simulink library "AEMS_Standard_Library"  (R2016b)
settings: Solver=ode45  StartTime=0.0  StopTime=10.0  RelTol=1e-3
undefined symbols (not defined in the file or in its folder): BkPY, carto, Cbx_extegr, Cbx_lpegrsys, Cbx_portegr, Cnx_bnk_nr_conf, Cnx_cyl_nr_conf, ConfigManagement, configuration_management, Cxx_dcm_io_tmr_end_xxxx, Cxx_dcm_rt_tmr_end, Cxx_DID_xxxx_IO_max, Cxx_DID_xxxx_IO_min, Cxx_egrhsofs, Cxx_vmaniegi, DEM_DEBOUNCE_FREEZE, DEM_DTR_CTL_INVISIBLE, DEM_DTR_CTL_NORMAL, Dem_DtrId2_XXX, Dem_DtrId3_XXX, Dem_DtrId4_XXX, Dem_DtrId5_XXX, Dem_DtrId6_XXX, Dem_DtrId7_XXX, Dem_DtrId8_XXX, Dem_DtrId9_XXX, Dem_DtrId_XXX, Dem_EnableConditionId2_XXX, Dem_EnableConditionId3_XXX, Dem_EnableConditionId4_XXX, Dem_EnableConditionId5_XXX, Dem_EnableConditionId6_XXX, Dem_EnableConditionId7_XXX, Dem_EnableConditionId8_XXX, Dem_EnableConditionId_XXX, Dem_EventId, Dem_EventId2_XXX, Dem_EventId3_XXX, Dem_EventId4_XXX, Dem_EventId5_XXX, Dem_EventId6_XXX, Dem_EventId7_XXX, Dem_EventId8_XXX, Dem_EventId9_XXX, Dem_EventId_Device_Faulttype, Dem_EventId_XXX, DEM_IUMPR_GENERAL_DENOMINATOR, DEM_OPCYC_IGNITION, Dem_RatioId2_XXX, Dem_RatioId3_XXX, Dem_RatioId4_XXX, Dem_RatioId5_XXX, Dem_RatioId6_XXX, Dem_RatioId7_XXX, Dem_RatioId8_XXX, Dem_RatioId_XXX, Dem_StorageConditionId2_XXX, Dem_StorageConditionId3_XXX, Dem_StorageConditionId4_XXX, Dem_StorageConditionId5_XXX ... (+65)
libraries: AEMS_Standard_Library x477, simulink x2
(part 25 of 39)

== system AEMS_Standard_Library/SUB/AEMS_DEM_TIME_BASED_DEBOUNCE_THRSHOLD_DYN_6D ==
  note: DemDebounceBehavior
  flag_set : Inport
  conditionfulfilled : Inport  Port=2
  prefailed : Inport  Port=3
  prepassed : Inport  Port=4
  reseteventdebounce : Inport  Port=5
  failedthreshold : Inport  Port=6
  passedthreshold : Inport  Port=7
  AEMS_DEM_TIME_BASED_DEBOUNCE_THRSHOLD_DYN_CALL1 : Subsystem
  AEMS_DEM_TIME_BASED_DEBOUNCE_THRSHOLD_DYN_CALL2 : Subsystem
  AEMS_DEM_TIME_BASED_DEBOUNCE_THRSHOLD_DYN_CALL3 : Subsystem
  AEMS_DEM_TIME_BASED_DEBOUNCE_THRSHOLD_DYN_CALL4 : Subsystem
  AEMS_DEM_TIME_BASED_DEBOUNCE_THRSHOLD_DYN_CALL5 : Subsystem
  AEMS_DEM_TIME_BASED_DEBOUNCE_THRSHOLD_DYN_CALL6 : Subsystem
  DemDebounceBehavior : Constant  Value=[0,0,0,0,0,0]  OutDataTypeStr=uint8
  Demux{,1..7} (8 alike) : Demux  Outputs=6
  Mux{1..4} (4 alike) : Mux  Inputs=6
  debouncevalue_for_failed : Outport
  debouncevalue_for_passed : Outport  Port=2
  failed : Outport  Port=3
  passed : Outport  Port=4
  wires:
  flag_set/1 -> Demux/1
  Demux/1 -> AEMS_DEM_TIME_BASED_DEBOUNCE_THRSHOLD_DYN_CALL1/Enable
  conditionfulfilled/1 -> Demux1/1  "conditionfulfilled"
  Demux1/1 -> AEMS_DEM_TIME_BASED_DEBOUNCE_THRSHOLD_DYN_CALL1/1(conditionfulfilled)
  Demux/2 -> AEMS_DEM_TIME_BASED_DEBOUNCE_THRSHOLD_DYN_CALL2/Enable
  Demux1/2 -> AEMS_DEM_TIME_BASED_DEBOUNCE_THRSHOLD_DYN_CALL2/1(conditionfulfilled)
  prefailed/1 -> Demux2/1  "prefailed"
  Demux2/1 -> AEMS_DEM_TIME_BASED_DEBOUNCE_THRSHOLD_DYN_CALL1/2(prefailed)
  Demux2/2 -> AEMS_DEM_TIME_BASED_DEBOUNCE_THRSHOLD_DYN_CALL2/2(prefailed)
  prepassed/1 -> Demux3/1  "prepassed"
  Demux3/1 -> AEMS_DEM_TIME_BASED_DEBOUNCE_THRSHOLD_DYN_CALL1/3(prepassed)
  Demux3/2 -> AEMS_DEM_TIME_BASED_DEBOUNCE_THRSHOLD_DYN_CALL2/3(prepassed)
  Demux4/1 -> AEMS_DEM_TIME_BASED_DEBOUNCE_THRSHOLD_DYN_CALL1/4(reseteventdebounce)
  reseteventdebounce/1 -> Demux4/1  "reseteventdebounce"
  Demux4/2 -> AEMS_DEM_TIME_BASED_DEBOUNCE_THRSHOLD_DYN_CALL2/4(reseteventdebounce)
  DemDebounceBehavior/1 -> Demux5/1  "behavior"
  Demux5/1 -> AEMS_DEM_TIME_BASED_DEBOUNCE_THRSHOLD_DYN_CALL1/5(DemDebounceBehavior)
  Demux5/2 -> AEMS_DEM_TIME_BASED_DEBOUNCE_THRSHOLD_DYN_CALL2/5(DemDebounceBehavior)
  Demux6/1 -> AEMS_DEM_TIME_BASED_DEBOUNCE_THRSHOLD_DYN_CALL1/6(DemCounterFailedThreshold)
  failedthreshold/1 -> Demux6/1  "failedthreshold"
  Demux6/2 -> AEMS_DEM_TIME_BASED_DEBOUNCE_THRSHOLD_DYN_CALL2/6(DemCounterFailedThreshold)
  Demux7/1 -> AEMS_DEM_TIME_BASED_DEBOUNCE_THRSHOLD_DYN_CALL1/7(DemCounterPassedThreshold)
  passedthreshold/1 -> Demux7/1  "passedthreshold"
  Demux7/2 -> AEMS_DEM_TIME_BASED_DEBOUNCE_THRSHOLD_DYN_CALL2/7(DemCounterPassedThreshold)
  Mux1/1 -> debouncevalue_for_failed/1
  AEMS_DEM_TIME_BASED_DEBOUNCE_THRSHOLD_DYN_CALL1/1(debouncevalue_for_failed) -> Mux1/1
  AEMS_DEM_TIME_BASED_DEBOUNCE_THRSHOLD_DYN_CALL2/1(debouncevalue_for_failed) -> Mux1/2
  Mux2/1 -> debouncevalue_for_passed/1
  AEMS_DEM_TIME_BASED_DEBOUNCE_THRSHOLD_DYN_CALL1/2(debouncevalue_for_passed) -> Mux2/1
  AEMS_DEM_TIME_BASED_DEBOUNCE_THRSHOLD_DYN_CALL2/2(debouncevalue_for_passed) -> Mux2/2
  Mux3/1 -> failed/1
  AEMS_DEM_TIME_BASED_DEBOUNCE_THRSHOLD_DYN_CALL1/3(failed) -> Mux3/1
  AEMS_DEM_TIME_BASED_DEBOUNCE_THRSHOLD_DYN_CALL2/3(failed) -> Mux3/2
  AEMS_DEM_TIME_BASED_DEBOUNCE_THRSHOLD_DYN_CALL1/4(passed) -> Mux4/1
  Mux4/1 -> passed/1
  AEMS_DEM_TIME_BASED_DEBOUNCE_THRSHOLD_DYN_CALL2/4(passed) -> Mux4/2
  Demux/3 -> AEMS_DEM_TIME_BASED_DEBOUNCE_THRSHOLD_DYN_CALL3/Enable
  Demux1/3 -> AEMS_DEM_TIME_BASED_DEBOUNCE_THRSHOLD_DYN_CALL3/1(conditionfulfilled)
  Demux2/3 -> AEMS_DEM_TIME_BASED_DEBOUNCE_THRSHOLD_DYN_CALL3/2(prefailed)
  Demux3/3 -> AEMS_DEM_TIME_BASED_DEBOUNCE_THRSHOLD_DYN_CALL3/3(prepassed)
  Demux4/3 -> AEMS_DEM_TIME_BASED_DEBOUNCE_THRSHOLD_DYN_CALL3/4(reseteventdebounce)
  Demux5/3 -> AEMS_DEM_TIME_BASED_DEBOUNCE_THRSHOLD_DYN_CALL3/5(DemDebounceBehavior)
  Demux6/3 -> AEMS_DEM_TIME_BASED_DEBOUNCE_THRSHOLD_DYN_CALL3/6(DemCounterFailedThreshold)
  Demux7/3 -> AEMS_DEM_TIME_BASED_DEBOUNCE_THRSHOLD_DYN_CALL3/7(DemCounterPassedThreshold)
  AEMS_DEM_TIME_BASED_DEBOUNCE_THRSHOLD_DYN_CALL3/1(debouncevalue_for_failed) -> Mux1/3
  AEMS_DEM_TIME_BASED_DEBOUNCE_THRSHOLD_DYN_CALL3/2(debouncevalue_for_passed) -> Mux2/3
  AEMS_DEM_TIME_BASED_DEBOUNCE_THRSHOLD_DYN_CALL3/3(failed) -> Mux3/3
  AEMS_DEM_TIME_BASED_DEBOUNCE_THRSHOLD_DYN_CALL3/4(passed) -> Mux4/3
  Demux/4 -> AEMS_DEM_TIME_BASED_DEBOUNCE_THRSHOLD_DYN_CALL4/Enable
  Demux1/4 -> AEMS_DEM_TIME_BASED_DEBOUNCE_THRSHOLD_DYN_CALL4/1(conditionfulfilled)
  Demux2/4 -> AEMS_DEM_TIME_BASED_DEBOUNCE_THRSHOLD_DYN_CALL4/2(prefailed)
  Demux3/4 -> AEMS_DEM_TIME_BASED_DEBOUNCE_THRSHOLD_DYN_CALL4/3(prepassed)
  Demux4/4 -> AEMS_DEM_TIME_BASED_DEBOUNCE_THRSHOLD_DYN_CALL4/4(reseteventdebounce)
  Demux5/4 -> AEMS_DEM_TIME_BASED_DEBOUNCE_THRSHOLD_DYN_CALL4/5(DemDebounceBehavior)
  Demux6/4 -> AEMS_DEM_TIME_BASED_DEBOUNCE_THRSHOLD_DYN_CALL4/6(DemCounterFailedThreshold)
  Demux7/4 -> AEMS_DEM_TIME_BASED_DEBOUNCE_THRSHOLD_DYN_CALL4/7(DemCounterPassedThreshold)
  AEMS_DEM_TIME_BASED_DEBOUNCE_THRSHOLD_DYN_CALL4/1(debouncevalue_for_failed) -> Mux1/4
  AEMS_DEM_TIME_BASED_DEBOUNCE_THRSHOLD_DYN_CALL4/2(debouncevalue_for_passed) -> Mux2/4
  AEMS_DEM_TIME_BASED_DEBOUNCE_THRSHOLD_DYN_CALL4/3(failed) -> Mux3/4
  AEMS_DEM_TIME_BASED_DEBOUNCE_THRSHOLD_DYN_CALL4/4(passed) -> Mux4/4
  Demux/5 -> AEMS_DEM_TIME_BASED_DEBOUNCE_THRSHOLD_DYN_CALL5/Enable
  Demux/6 -> AEMS_DEM_TIME_BASED_DEBOUNCE_THRSHOLD_DYN_CALL6/Enable
  Demux1/5 -> AEMS_DEM_TIME_BASED_DEBOUNCE_THRSHOLD_DYN_CALL5/1(conditionfulfilled)
  Demux1/6 -> AEMS_DEM_TIME_BASED_DEBOUNCE_THRSHOLD_DYN_CALL6/1(conditionfulfilled)
  Demux2/5 -> AEMS_DEM_TIME_BASED_DEBOUNCE_THRSHOLD_DYN_CALL5/2(prefailed)
  Demux2/6 -> AEMS_DEM_TIME_BASED_DEBOUNCE_THRSHOLD_DYN_CALL6/2(prefailed)
  Demux3/5 -> AEMS_DEM_TIME_BASED_DEBOUNCE_THRSHOLD_DYN_CALL5/3(prepassed)
  Demux3/6 -> AEMS_DEM_TIME_BASED_DEBOUNCE_THRSHOLD_DYN_CALL6/3(prepassed)
  Demux4/5 -> AEMS_DEM_TIME_BASED_DEBOUNCE_THRSHOLD_DYN_CALL5/4(reseteventdebounce)
  Demux4/6 -> AEMS_DEM_TIME_BASED_DEBOUNCE_THRSHOLD_DYN_CALL6/4(reseteventdebounce)
  Demux5/5 -> AEMS_DEM_TIME_BASED_DEBOUNCE_THRSHOLD_DYN_CALL5/5(DemDebounceBehavior)
  Demux5/6 -> AEMS_DEM_TIME_BASED_DEBOUNCE_THRSHOLD_DYN_CALL6/5(DemDebounceBehavior)
  Demux6/5 -> AEMS_DEM_TIME_BASED_DEBOUNCE_THRSHOLD_DYN_CALL5/6(DemCounterFailedThreshold)
  Demux6/6 -> AEMS_DEM_TIME_BASED_DEBOUNCE_THRSHOLD_DYN_CALL6/6(DemCounterFailedThreshold)
  Demux7/5 -> AEMS_DEM_TIME_BASED_DEBOUNCE_THRSHOLD_DYN_CALL5/7(DemCounterPassedThreshold)
  Demux7/6 -> AEMS_DEM_TIME_BASED_DEBOUNCE_THRSHOLD_DYN_CALL6/7(DemCounterPassedThreshold)
  AEMS_DEM_TIME_BASED_DEBOUNCE_THRSHOLD_DYN_CALL5/1(debouncevalue_for_failed) -> Mux1/5
  AEMS_DEM_TIME_BASED_DEBOUNCE_THRSHOLD_DYN_CALL6/1(debouncevalue_for_failed) -> Mux1/6
  AEMS_DEM_TIME_BASED_DEBOUNCE_THRSHOLD_DYN_CALL5/2(debouncevalue_for_passed) -> Mux2/5
  AEMS_DEM_TIME_BASED_DEBOUNCE_THRSHOLD_DYN_CALL6/2(debouncevalue_for_passed) -> Mux2/6
  AEMS_DEM_TIME_BASED_DEBOUNCE_THRSHOLD_DYN_CALL5/3(failed) -> Mux3/5
  AEMS_DEM_TIME_BASED_DEBOUNCE_THRSHOLD_DYN_CALL6/3(failed) -> Mux3/6
  AEMS_DEM_TIME_BASED_DEBOUNCE_THRSHOLD_DYN_CALL5/4(passed) -> Mux4/5
  AEMS_DEM_TIME_BASED_DEBOUNCE_THRSHOLD_DYN_CALL6/4(passed) -> Mux4/6

== system AEMS_Standard_Library/SUB/AEMS_DEM_TIME_BASED_DEBOUNCE_THRSHOLD_DYN_8D ==
  note: DemDebounceBehavior
  flag_set : Inport
  conditionfulfilled : Inport  Port=2
  prefailed : Inport  Port=3
  prepassed : Inport  Port=4
  reseteventdebounce : Inport  Port=5
  failedthreshold : Inport  Port=6
  passedthreshold : Inport  Port=7
  AEMS_DEM_TIME_BASED_DEBOUNCE_THRSHOLD_DYN_CALL1 : Subsystem
  AEMS_DEM_TIME_BASED_DEBOUNCE_THRSHOLD_DYN_CALL2 : Subsystem
  AEMS_DEM_TIME_BASED_DEBOUNCE_THRSHOLD_DYN_CALL3 : Subsystem
  AEMS_DEM_TIME_BASED_DEBOUNCE_THRSHOLD_DYN_CALL4 : Subsystem
  AEMS_DEM_TIME_BASED_DEBOUNCE_THRSHOLD_DYN_CALL5 : Subsystem
  AEMS_DEM_TIME_BASED_DEBOUNCE_THRSHOLD_DYN_CALL6 : Subsystem
  AEMS_DEM_TIME_BASED_DEBOUNCE_THRSHOLD_DYN_CALL7 : Subsystem
  AEMS_DEM_TIME_BASED_DEBOUNCE_THRSHOLD_DYN_CALL8 : Subsystem
  DemDebounceBehavior : Constant  Value=[0,0,0,0,0,0,0,0]  OutDataTypeStr=uint8
  Demux{,1..7} (8 alike) : Demux  Outputs=8
  Mux{1..4} (4 alike) : Mux  Inputs=8
  debouncevalue_for_failed : Outport
  debouncevalue_for_passed : Outport  Port=2
  failed : Outport  Port=3
  passed : Outport  Port=4
  wires:
  flag_set/1 -> Demux/1
  Demux/1 -> AEMS_DEM_TIME_BASED_DEBOUNCE_THRSHOLD_DYN_CALL1/Enable
  conditionfulfilled/1 -> Demux1/1  "conditionfulfilled"
  Demux1/1 -> AEMS_DEM_TIME_BASED_DEBOUNCE_THRSHOLD_DYN_CALL1/1(conditionfulfilled)
  Demux/2 -> AEMS_DEM_TIME_BASED_DEBOUNCE_THRSHOLD_DYN_CALL2/Enable
  Demux1/2 -> AEMS_DEM_TIME_BASED_DEBOUNCE_THRSHOLD_DYN_CALL2/1(conditionfulfilled)
  prefailed/1 -> Demux2/1  "prefailed"
  Demux2/1 -> AEMS_DEM_TIME_BASED_DEBOUNCE_THRSHOLD_DYN_CALL1/2(prefailed)
  Demux2/2 -> AEMS_DEM_TIME_BASED_DEBOUNCE_THRSHOLD_DYN_CALL2/2(prefailed)
  prepassed/1 -> Demux3/1  "prepassed"
  Demux3/1 -> AEMS_DEM_TIME_BASED_DEBOUNCE_THRSHOLD_DYN_CALL1/3(prepassed)
  Demux3/2 -> AEMS_DEM_TIME_BASED_DEBOUNCE_THRSHOLD_DYN_CALL2/3(prepassed)
  Demux4/1 -> AEMS_DEM_TIME_BASED_DEBOUNCE_THRSHOLD_DYN_CALL1/4(reseteventdebounce)
  reseteventdebounce/1 -> Demux4/1  "reseteventdebounce"
  Demux4/2 -> AEMS_DEM_TIME_BASED_DEBOUNCE_THRSHOLD_DYN_CALL2/4(reseteventdebounce)
  DemDebounceBehavior/1 -> Demux5/1  "behavior"
  Demux5/1 -> AEMS_DEM_TIME_BASED_DEBOUNCE_THRSHOLD_DYN_CALL1/5(DemDebounceBehavior)
  Demux5/2 -> AEMS_DEM_TIME_BASED_DEBOUNCE_THRSHOLD_DYN_CALL2/5(DemDebounceBehavior)
  Demux6/1 -> AEMS_DEM_TIME_BASED_DEBOUNCE_THRSHOLD_DYN_CALL1/6(DemCounterFailedThreshold)
  failedthreshold/1 -> Demux6/1  "failedthreshold"
  Demux6/2 -> AEMS_DEM_TIME_BASED_DEBOUNCE_THRSHOLD_DYN_CALL2/6(DemCounterFailedThreshold)
  Demux7/1 -> AEMS_DEM_TIME_BASED_DEBOUNCE_THRSHOLD_DYN_CALL1/7(DemCounterPassedThreshold)
  passedthreshold/1 -> Demux7/1  "passedthreshold"
  Demux7/2 -> AEMS_DEM_TIME_BASED_DEBOUNCE_THRSHOLD_DYN_CALL2/7(DemCounterPassedThreshold)
  Mux1/1 -> debouncevalue_for_failed/1
  AEMS_DEM_TIME_BASED_DEBOUNCE_THRSHOLD_DYN_CALL1/1(debouncevalue_for_failed) -> Mux1/1
  AEMS_DEM_TIME_BASED_DEBOUNCE_THRSHOLD_DYN_CALL2/1(debouncevalue_for_failed) -> Mux1/2
  Mux2/1 -> debouncevalue_for_passed/1
  AEMS_DEM_TIME_BASED_DEBOUNCE_THRSHOLD_DYN_CALL1/2(debouncevalue_for_passed) -> Mux2/1
  AEMS_DEM_TIME_BASED_DEBOUNCE_THRSHOLD_DYN_CALL2/2(debouncevalue_for_passed) -> Mux2/2
  Mux3/1 -> failed/1
  AEMS_DEM_TIME_BASED_DEBOUNCE_THRSHOLD_DYN_CALL1/3(failed) -> Mux3/1
  AEMS_DEM_TIME_BASED_DEBOUNCE_THRSHOLD_DYN_CALL2/3(failed) -> Mux3/2
  AEMS_DEM_TIME_BASED_DEBOUNCE_THRSHOLD_DYN_CALL1/4(passed) -> Mux4/1
  Mux4/1 -> passed/1
  AEMS_DEM_TIME_BASED_DEBOUNCE_THRSHOLD_DYN_CALL2/4(passed) -> Mux4/2
  Demux/3 -> AEMS_DEM_TIME_BASED_DEBOUNCE_THRSHOLD_DYN_CALL3/Enable
  Demux1/3 -> AEMS_DEM_TIME_BASED_DEBOUNCE_THRSHOLD_DYN_CALL3/1(conditionfulfilled)
  Demux2/3 -> AEMS_DEM_TIME_BASED_DEBOUNCE_THRSHOLD_DYN_CALL3/2(prefailed)
  Demux3/3 -> AEMS_DEM_TIME_BASED_DEBOUNCE_THRSHOLD_DYN_CALL3/3(prepassed)
  Demux4/3 -> AEMS_DEM_TIME_BASED_DEBOUNCE_THRSHOLD_DYN_CALL3/4(reseteventdebounce)
  Demux5/3 -> AEMS_DEM_TIME_BASED_DEBOUNCE_THRSHOLD_DYN_CALL3/5(DemDebounceBehavior)
  Demux6/3 -> AEMS_DEM_TIME_BASED_DEBOUNCE_THRSHOLD_DYN_CALL3/6(DemCounterFailedThreshold)
  Demux7/3 -> AEMS_DEM_TIME_BASED_DEBOUNCE_THRSHOLD_DYN_CALL3/7(DemCounterPassedThreshold)
  AEMS_DEM_TIME_BASED_DEBOUNCE_THRSHOLD_DYN_CALL3/1(debouncevalue_for_failed) -> Mux1/3
  AEMS_DEM_TIME_BASED_DEBOUNCE_THRSHOLD_DYN_CALL3/2(debouncevalue_for_passed) -> Mux2/3
  AEMS_DEM_TIME_BASED_DEBOUNCE_THRSHOLD_DYN_CALL3/3(failed) -> Mux3/3
  AEMS_DEM_TIME_BASED_DEBOUNCE_THRSHOLD_DYN_CALL3/4(passed) -> Mux4/3
  Demux/4 -> AEMS_DEM_TIME_BASED_DEBOUNCE_THRSHOLD_DYN_CALL4/Enable
  Demux1/4 -> AEMS_DEM_TIME_BASED_DEBOUNCE_THRSHOLD_DYN_CALL4/1(conditionfulfilled)
  Demux2/4 -> AEMS_DEM_TIME_BASED_DEBOUNCE_THRSHOLD_DYN_CALL4/2(prefailed)
  Demux3/4 -> AEMS_DEM_TIME_BASED_DEBOUNCE_THRSHOLD_DYN_CALL4/3(prepassed)
  Demux4/4 -> AEMS_DEM_TIME_BASED_DEBOUNCE_THRSHOLD_DYN_CALL4/4(reseteventdebounce)
  Demux5/4 -> AEMS_DEM_TIME_BASED_DEBOUNCE_THRSHOLD_DYN_CALL4/5(DemDebounceBehavior)
  Demux6/4 -> AEMS_DEM_TIME_BASED_DEBOUNCE_THRSHOLD_DYN_CALL4/6(DemCounterFailedThreshold)
  Demux7/4 -> AEMS_DEM_TIME_BASED_DEBOUNCE_THRSHOLD_DYN_CALL4/7(DemCounterPassedThreshold)
  AEMS_DEM_TIME_BASED_DEBOUNCE_THRSHOLD_DYN_CALL4/1(debouncevalue_for_failed) -> Mux1/4
  AEMS_DEM_TIME_BASED_DEBOUNCE_THRSHOLD_DYN_CALL4/2(debouncevalue_for_passed) -> Mux2/4
  AEMS_DEM_TIME_BASED_DEBOUNCE_THRSHOLD_DYN_CALL4/3(failed) -> Mux3/4
  AEMS_DEM_TIME_BASED_DEBOUNCE_THRSHOLD_DYN_CALL4/4(passed) -> Mux4/4
  Demux/5 -> AEMS_DEM_TIME_BASED_DEBOUNCE_THRSHOLD_DYN_CALL5/Enable
  Demux/6 -> AEMS_DEM_TIME_BASED_DEBOUNCE_THRSHOLD_DYN_CALL6/Enable
  Demux1/5 -> AEMS_DEM_TIME_BASED_DEBOUNCE_THRSHOLD_DYN_CALL5/1(conditionfulfilled)
  Demux1/6 -> AEMS_DEM_TIME_BASED_DEBOUNCE_THRSHOLD_DYN_CALL6/1(conditionfulfilled)
  Demux2/5 -> AEMS_DEM_TIME_BASED_DEBOUNCE_THRSHOLD_DYN_CALL5/2(prefailed)
  Demux2/6 -> AEMS_DEM_TIME_BASED_DEBOUNCE_THRSHOLD_DYN_CALL6/2(prefailed)
  Demux3/5 -> AEMS_DEM_TIME_BASED_DEBOUNCE_THRSHOLD_DYN_CALL5/3(prepassed)
  Demux3/6 -> AEMS_DEM_TIME_BASED_DEBOUNCE_THRSHOLD_DYN_CALL6/3(prepassed)
  Demux4/5 -> AEMS_DEM_TIME_BASED_DEBOUNCE_THRSHOLD_DYN_CALL5/4(reseteventdebounce)
  Demux4/6 -> AEMS_DEM_TIME_BASED_DEBOUNCE_THRSHOLD_DYN_CALL6/4(reseteventdebounce)
  Demux5/5 -> AEMS_DEM_TIME_BASED_DEBOUNCE_THRSHOLD_DYN_CALL5/5(DemDebounceBehavior)
  Demux5/6 -> AEMS_DEM_TIME_BASED_DEBOUNCE_THRSHOLD_DYN_CALL6/5(DemDebounceBehavior)
  Demux6/5 -> AEMS_DEM_TIME_BASED_DEBOUNCE_THRSHOLD_DYN_CALL5/6(DemCounterFailedThreshold)
  Demux6/6 -> AEMS_DEM_TIME_BASED_DEBOUNCE_THRSHOLD_DYN_CALL6/6(DemCounterFailedThreshold)
  Demux7/5 -> AEMS_DEM_TIME_BASED_DEBOUNCE_THRSHOLD_DYN_CALL5/7(DemCounterPassedThreshold)
  Demux7/6 -> AEMS_DEM_TIME_BASED_DEBOUNCE_THRSHOLD_DYN_CALL6/7(DemCounterPassedThreshold)
  AEMS_DEM_TIME_BASED_DEBOUNCE_THRSHOLD_DYN_CALL5/1(debouncevalue_for_failed) -> Mux1/5
  AEMS_DEM_TIME_BASED_DEBOUNCE_THRSHOLD_DYN_CALL6/1(debouncevalue_for_failed) -> Mux1/6
  AEMS_DEM_TIME_BASED_DEBOUNCE_THRSHOLD_DYN_CALL5/2(debouncevalue_for_passed) -> Mux2/5
  AEMS_DEM_TIME_BASED_DEBOUNCE_THRSHOLD_DYN_CALL6/2(debouncevalue_for_passed) -> Mux2/6
  AEMS_DEM_TIME_BASED_DEBOUNCE_THRSHOLD_DYN_CALL5/3(failed) -> Mux3/5
  AEMS_DEM_TIME_BASED_DEBOUNCE_THRSHOLD_DYN_CALL6/3(failed) -> Mux3/6
  AEMS_DEM_TIME_BASED_DEBOUNCE_THRSHOLD_DYN_CALL5/4(passed) -> Mux4/5
  AEMS_DEM_TIME_BASED_DEBOUNCE_THRSHOLD_DYN_CALL6/4(passed) -> Mux4/6
  Demux/7 -> AEMS_DEM_TIME_BASED_DEBOUNCE_THRSHOLD_DYN_CALL7/Enable
  Demux/8 -> AEMS_DEM_TIME_BASED_DEBOUNCE_THRSHOLD_DYN_CALL8/Enable
  Demux1/7 -> AEMS_DEM_TIME_BASED_DEBOUNCE_THRSHOLD_DYN_CALL7/1(conditionfulfilled)
  Demux1/8 -> AEMS_DEM_TIME_BASED_DEBOUNCE_THRSHOLD_DYN_CALL8/1(conditionfulfilled)
  Demux2/7 -> AEMS_DEM_TIME_BASED_DEBOUNCE_THRSHOLD_DYN_CALL7/2(prefailed)
  Demux2/8 -> AEMS_DEM_TIME_BASED_DEBOUNCE_THRSHOLD_DYN_CALL8/2(prefailed)
  Demux3/7 -> AEMS_DEM_TIME_BASED_DEBOUNCE_THRSHOLD_DYN_CALL7/3(prepassed)
  Demux3/8 -> AEMS_DEM_TIME_BASED_DEBOUNCE_THRSHOLD_DYN_CALL8/3(prepassed)
  Demux4/7 -> AEMS_DEM_TIME_BASED_DEBOUNCE_THRSHOLD_DYN_CALL7/4(reseteventdebounce)
  Demux4/8 -> AEMS_DEM_TIME_BASED_DEBOUNCE_THRSHOLD_DYN_CALL8/4(reseteventdebounce)
  Demux5/7 -> AEMS_DEM_TIME_BASED_DEBOUNCE_THRSHOLD_DYN_CALL7/5(DemDebounceBehavior)
  Demux5/8 -> AEMS_DEM_TIME_BASED_DEBOUNCE_THRSHOLD_DYN_CALL8/5(DemDebounceBehavior)
  Demux6/7 -> AEMS_DEM_TIME_BASED_DEBOUNCE_THRSHOLD_DYN_CALL7/6(DemCounterFailedThreshold)
  Demux6/8 -> AEMS_DEM_TIME_BASED_DEBOUNCE_THRSHOLD_DYN_CALL8/6(DemCounterFailedThreshold)
  Demux7/7 -> AEMS_DEM_TIME_BASED_DEBOUNCE_THRSHOLD_DYN_CALL7/7(DemCounterPassedThreshold)
  Demux7/8 -> AEMS_DEM_TIME_BASED_DEBOUNCE_THRSHOLD_DYN_CALL8/7(DemCounterPassedThreshold)
  AEMS_DEM_TIME_BASED_DEBOUNCE_THRSHOLD_DYN_CALL7/1(debouncevalue_for_failed) -> Mux1/7
  AEMS_DEM_TIME_BASED_DEBOUNCE_THRSHOLD_DYN_CALL8/1(debouncevalue_for_failed) -> Mux1/8
  AEMS_DEM_TIME_BASED_DEBOUNCE_THRSHOLD_DYN_CALL7/2(debouncevalue_for_passed) -> Mux2/7
  AEMS_DEM_TIME_BASED_DEBOUNCE_THRSHOLD_DYN_CALL8/2(debouncevalue_for_passed) -> Mux2/8
  AEMS_DEM_TIME_BASED_DEBOUNCE_THRSHOLD_DYN_CALL7/3(failed) -> Mux3/7
  AEMS_DEM_TIME_BASED_DEBOUNCE_THRSHOLD_DYN_CALL8/3(failed) -> Mux3/8
  AEMS_DEM_TIME_BASED_DEBOUNCE_THRSHOLD_DYN_CALL7/4(passed) -> Mux4/7
  AEMS_DEM_TIME_BASED_DEBOUNCE_THRSHOLD_DYN_CALL8/4(passed) -> Mux4/8

== system AEMS_Standard_Library/SUB/AEMS_FIM_GETFUNCTIONPERMISSION ==
  fid : Inport
  Data Type Conversion : DataTypeConversion  SaturateOnIntegerOverflow=on
  Data Type Conversion1 : DataTypeConversion  OutDataTypeStr=uint8
  Ground1 : Ground
  Source_Of_Permission_Port : Constant  OutDataTypeStr=boolean
  Terminator : Terminator
  Terminator1 : Terminator
  permission : Outport
  wires:
  Source_Of_Permission_Port/1 -> Data Type Conversion/1
  Data Type Conversion/1 -> permission/1  "permission"
  fid/1 -> Terminator/1
  Ground1/1 -> Data Type Conversion1/1
  Data Type Conversion1/1 -> Terminator1/1  "Std_ReturnType"

== system AEMS_Standard_Library/SUB/AEMS_FIM_GET_FUNC_PMT_1D ==
  AEMS_FIM_GETFUNCTIONPERMISSION : AEMS_Standard_Library/SUB/AEMS_FIM_GETFUNCTIONPERMISSION  Tag=[LIB]  FID=Fim_fid_xxxx  FunctionMode=Functional
      settings: AttributesFormatString=%<MaskType>\nFunction Mode = %<FunctionMode>\nDowngraded mode short name : = %<FID>
  FID_Block : Constant  Value=Fim_fid_xxxx  OutDataTypeStr=uint8
  not : Logic  Operator=NOT  Inputs=1  OutDataTypeStr=boolean
  permission_flag : Outport
  wires:
  AEMS_FIM_GETFUNCTIONPERMISSION/1 -> not/1
  FID_Block/1 -> AEMS_FIM_GETFUNCTIONPERMISSION/1
  not/1 -> permission_flag/1  "permission_flag"

== system AEMS_Standard_Library/SUB/AEMS_FIM_GET_FUNC_PMT_2D ==
  AEMS_FIM_GETFUNCTIONPERMISSION : AEMS_Standard_Library/SUB/AEMS_FIM_GETFUNCTIONPERMISSION  Tag=[LIB]  FID=Fim_fid_xxxx_1  FunctionMode=Functional
      settings: AttributesFormatString=%<MaskType>\nFunction Mode = %<FunctionMode>\nDowngraded mode short name : = %<FID>
  AEMS_FIM_GETFUNCTIONPERMISSION1 : AEMS_Standard_Library/SUB/AEMS_FIM_GETFUNCTIONPERMISSION  Tag=[LIB]  FID=Fim_fid_xxxx_2  FunctionMode=Functional
      settings: AttributesFormatString=%<MaskType>\nFunction Mode = %<FunctionMode>\nDowngraded mode short name : = %<FID>
  Data Type Conversion : DataTypeConversion  OutDataTypeStr=boolean  SaturateOnIntegerOverflow=on
  FID_Block1 : Constant  Value=Fim_fid_xxxx_1  OutDataTypeStr=uint8
  FID_Block2 : Constant  Value=Fim_fid_xxxx_2  OutDataTypeStr=uint8
  Mux : Mux  Inputs=2
  not : Logic  Operator=NOT  Inputs=1  OutDataTypeStr=boolean
  not1 : Logic  Operator=NOT  Inputs=1  OutDataTypeStr=boolean
  permission_flag : Outport
  wires:
  not/1 -> Mux/1  "permission_flag1"
  FID_Block1/1 -> AEMS_FIM_GETFUNCTIONPERMISSION/1
  not1/1 -> Mux/2  "permission_flag2"
  FID_Block2/1 -> AEMS_FIM_GETFUNCTIONPERMISSION1/1
  Mux/1 -> Data Type Conversion/1
  Data Type Conversion/1 -> permission_flag/1  "permission_flag"
  AEMS_FIM_GETFUNCTIONPERMISSION/1 -> not/1
  AEMS_FIM_GETFUNCTIONPERMISSION1/1 -> not1/1

== system AEMS_Standard_Library/SUB/AEMS_SORT_MEDIAN ==
  Sorted_vector : Inport
  Vector_size : Inport  Port=2
  Constant3 : Constant  Value=2  OutDataTypeStr=uint8
  If : If  IfExpression=u1 ~= 0
  Math Function : Math  Operator=mod  SaturateOnIntegerOverflow=on
  Merge : Merge  InitialOutput=0
      settings: AttributesFormatString=<initial=%<InitialOutput>>
  Odd : Subsystem  TreatAsAtomicUnit=on
  Pair : Subsystem  TreatAsAtomicUnit=on
  Median_Vector : Outport
  wires:
  Constant3/1 -> Math Function/2
  Math Function/1 -> If/1
  Vector_size/1 -> Odd/1(Vector_size), Pair/1(Vector_size), Math Function/1
  If/1 -> Pair/Action
  If/2 -> Odd/Action
  Pair/1(Median_Pair) -> Merge/1
  Odd/1(Median_Odd) -> Merge/2
  Merge/1 -> Median_Vector/1
  Sorted_vector/1 -> Odd/2(Sorted_vector), Pair/2(Sorted_vector)

== system AEMS_Standard_Library/TIMER/AEMS_SW_TIMER2 ==
  note: Time
  note: Flag 1
  note: Flag 1
  note: Time Inc++
  note: Flag 2
  note: Time
  note: Flag has been set in every State to identify the previous State and muxed with output(Time).
      | Flag 1- TIMER/
      | Flag 2 - ARRET
  note: State - TIMER/
  Start : Inport
  Stop : Inport  Port=2
  Timestep : Inport  Port=3
  BusCreator : BusCreator  Inputs=2
  BusCreator1 : BusCreator  Inputs=2
  BusCreator2 : BusCreator  Inputs=2
  BusSelector : BusSelector  OutputSignals=signal2,signal1
  Constant1 : Constant  Tag=AM,Constant,0,1,Value;CMP,Value;  Value=1000  OutDataTypeStr=Inherit: Inherit via back propagation
  Constant10 : Constant  Value=0  OutDataTypeStr=Inherit: Inherit via back propagation
  Constant13 : Constant  OutDataTypeStr=uint8
  Constant14 : Constant  Value=0  OutDataTypeStr=Inherit: Inherit via back propagation
  Constant15 : Constant  Value=2  OutDataTypeStr=uint8
  Constant19 : Constant  OutDataTypeStr=uint8
  Constant2 : Constant  Tag=AM,Constant,0,1,Value;CMP,Value;  Value=1000  OutDataTypeStr=Inherit: Inherit via back propagation
  Divide1 : Product  Inputs=*/  OutDataTypeStr=Inherit: Inherit via back propagation  RndMeth=Zero
      settings: AttributesFormatString=SAT = %<SaturateOnIntegerOverflow>
  MultiportSwitch : MultiPortSwitch  DataPortOrder=Zero-based contiguous  zeroidx=on  RndMeth=Zero  InputSameDT=on
      settings: AttributesFormatString=PortOrder=%<DataPortOrder>
  Product2 : Product  OutDataTypeStr=Inherit: Inherit via back propagation  RndMeth=Zero
      settings: AttributesFormatString=SAT = %<SaturateOnIntegerOverflow>
  Subtract1 : Sum  OutDataTypeStr=Inherit: Inherit via back propagation  RndMeth=Zero  InputSameDT=on
  Switch3 : Switch  Criteria=u2 ~= 0  RndMeth=Zero  InputSameDT=on
      settings: AttributesFormatString=Criteria=%<Criteria>
  Switch5 : Switch  Criteria=u2 ~= 0  RndMeth=Zero  InputSameDT=on
      settings: AttributesFormatString=Criteria=%<Criteria>
  UnitDelay : UnitDelay  SampleTime=-1
      settings: AttributesFormatString=IC = %<X0>
  UnitDelay1 : UnitDelay  SampleTime=-1
      settings: AttributesFormatString=IC = %<X0>
  Time : Outport  InitialOutput=0
  wires:
  Divide1/1 -> Time/1
  BusSelector/2 -> Divide1/1, UnitDelay1/1  "<signal1>"
  UnitDelay1/1 -> Subtract1/1
  BusSelector/1 -> UnitDelay/1  "<signal2>"
  MultiportSwitch/1 -> BusSelector/1
  Start/1 -> Switch3/2
  Constant10/1 -> BusCreator/1
  Constant13/1 -> BusCreator/2
  BusCreator/1 -> Switch3/1
  Constant14/1 -> BusCreator1/1
  Constant15/1 -> BusCreator1/2
  Switch3/1 -> MultiportSwitch/2, MultiportSwitch/4
  UnitDelay/1 -> MultiportSwitch/1
  Stop/1 -> Switch5/2
  Constant19/1 -> BusCreator2/2
  Subtract1/1 -> BusCreator2/1
  BusCreator2/1 -> Switch5/3
  Switch5/1 -> MultiportSwitch/3
  BusCreator1/1 -> Switch3/3, Switch5/1
  Product2/1 -> Subtract1/2
  Timestep/1 -> Product2/1
  Constant2/1 -> Product2/2
  Constant1/1 -> Divide1/2

== system AEMS_Standard_Library/TIMER/AEMS_SW_TIMER_INIT ==
  Enable : Inport  Tag=AM,In,0,1,Name,C;CMP,Port,PortWidth,SampleTime;
  Init : Inport  Tag=AM,In,0,1,Name,C;CMP,Port,PortWidth,SampleTime;  Port=2
  Timestep : Inport  Tag=AM,In,0,1,Name,C;CMP,Port,PortWidth,SampleTime;  Port=3
  Constant1 : Constant  Tag=AM,Constant,0,1,Value;CMP,Value;  Value=1000  OutDataTypeStr=Inherit: Inherit via back propagation
  Constant2 : Constant  Tag=AM,Constant,0,1,Value;CMP,Value;  Value=1000  OutDataTypeStr=Inherit: Inherit via back propagation
  Divide1 : Product  Inputs=*/  OutDataTypeStr=Inherit: Inherit via back propagation  RndMeth=Zero
  Logical_Operator : Logic  OutDataTypeStr=boolean
  Logical_Operator1 : Logic  OutDataTypeStr=boolean
  Logical_Operator2 : Logic  Operator=NOT  OutDataTypeStr=boolean
  Logical_Operator3 : Logic  Operator=OR  OutDataTypeStr=boolean
  Logical_Operator4 : Logic  Operator=OR  OutDataTypeStr=boolean
  Logical_Operator5 : Logic  Operator=OR  OutDataTypeStr=boolean
  Logical_Operator6 : Logic  Operator=NOT  OutDataTypeStr=boolean
  Product2 : Product  OutDataTypeStr=Inherit: Inherit via back propagation  RndMeth=Zero
  Sum1 : Sum  OutDataTypeStr=Inherit: Inherit via back propagation  RndMeth=Zero  InputSameDT=on
  Switch : Switch  Tag=GEN,Threshold;AM,Switch,2,1;CMP,Threshold;  Criteria=u2 ~= 0  RndMeth=Zero  SaturateOnIntegerOverflow=on  InputSameDT=on
      settings: AttributesFormatString=Criteria=%<Criteria>
  Switch2 : Switch  Tag=GEN,Threshold;AM,Switch,2,1;CMP,Threshold;  Criteria=u2 ~= 0  RndMeth=Zero  SaturateOnIntegerOverflow=on  InputSameDT=on
      settings: AttributesFormatString=Criteria=%<Criteria>
  Unit_Delay : UnitDelay  Description=\nStore in Global RAM  SampleTime=-1
      settings: AttributesFormatString=IC = %<X0>
  Unit_Delay2 : UnitDelay  Description=\nStore in Global RAM  InitialCondition=false  SampleTime=-1
      settings: AttributesFormatString=IC = %<X0>
  Unit_Delay3 : UnitDelay  Description=\nStore in Global RAM  InitialCondition=false  SampleTime=-1
      settings: AttributesFormatString=IC = %<X0>
  Unit_Delay7 : UnitDelay  Description=\nStore in Global RAM  SampleTime=-1
      settings: AttributesFormatString=IC = %<X0>
  Unit_Delay8 : UnitDelay  Description=\nStore in Global RAM  SampleTime=-1
      settings: AttributesFormatString=IC = %<X0>
  imm_zero : Constant  Tag=AM,Constant,0,1,Value;CMP,Value;  Value=0  OutDataTypeStr=Inherit: Inherit via back propagation
  imm_zero1 : Constant  Tag=AM,Constant,0,1,Value;CMP,Value;  Value=true  OutDataTypeStr=Inherit: Inherit via back propagation
  Time : Outport  Tag=AM,Out,1,0,Name,NC;CMP,Port,OutputWhenDisabled,InitialOutput;
  wires:
  Constant1/1 -> Product2/2
  Constant2/1 -> Divide1/2
  imm_zero/1 -> Switch/1
  Switch/1 -> Divide1/1, Unit_Delay/1
  Unit_Delay/1 -> Sum1/2, Switch2/3
  Sum1/1 -> Switch2/1
  Switch2/1 -> Switch/3
  Enable/1 -> Unit_Delay7/1, Logical_Operator1/1
  imm_zero1/1 -> Unit_Delay2/1
  Unit_Delay2/1 -> Unit_Delay3/1
  Unit_Delay7/1 -> Logical_Operator5/1, Logical_Operator2/1
  Logical_Operator2/1 -> Logical_Operator3/1
  Logical_Operator3/1 -> Logical_Operator/2
  Logical_Operator/1 -> Logical_Operator4/1
  Logical_Operator4/1 -> Switch/2
  Unit_Delay3/1 -> Logical_Operator6/1
  Init/1 -> Logical_Operator4/2, Unit_Delay8/1
  Unit_Delay8/1 -> Logical_Operator3/2, Logical_Operator5/2
  Logical_Operator5/1 -> Logical_Operator1/2
  Logical_Operator1/1 -> Switch2/2
  Timestep/1 -> Product2/1
  Divide1/1 -> Time/1
  Product2/1 -> Sum1/1
  Logical_Operator6/1 -> Logical_Operator/1

== system AEMS_Standard_Library/TIMER/AEMS_TIMER ==
  start_flag : Inport  OutDataTypeStr=boolean
  target_time : Inport  Port=2
  Constant1 : Constant  Value=sample_time  OutDataTypeStr=single
  Constant3 : Constant  Value=0.0001  OutDataTypeStr=single
  Constant5 : Constant  Value=0  OutDataTypeStr=Inherit: Inherit via back propagation
  Logical Operator1 : Logic  Operator=NOT  OutDataTypeStr=boolean
  Logical Operator2 : Logic  OutDataTypeStr=boolean
  Logical Operator4 : Logic  Operator=NOT  OutDataTypeStr=boolean
  Logical Operator5 : Logic  OutDataTypeStr=boolean
  Logical Operator7 : Logic  Operator=OR  OutDataTypeStr=boolean
  MinMax : MinMax  Inputs=2  SaturateOnIntegerOverflow=on  InputSameDT=on
  Relational Operator : RelationalOperator  Operator=<=  OutDataTypeStr=boolean  RndMeth=Nearest  InputSameDT=on
  Sum : Sum  OutDataTypeStr=single  SaturateOnIntegerOverflow=on
  Sum1 : Sum  SaturateOnIntegerOverflow=on
  Switch2 : Switch  Criteria=u2 ~= 0  SaturateOnIntegerOverflow=on  InputSameDT=on
      settings: AttributesFormatString=Criteria=%<Criteria>
  Switch3 : Switch  Criteria=u2 ~= 0  SaturateOnIntegerOverflow=on  InputSameDT=on
      settings: AttributesFormatString=Criteria=%<Criteria>
  Unit Delay : UnitDelay  SampleTime=-1
      settings: AttributesFormatString=<initial=%<InitialCondition>>
  Unit Delay1 : UnitDelay  SampleTime=-1
      settings: AttributesFormatString=<initial=%<InitialCondition>>
  Unit Delay2 : UnitDelay  SampleTime=-1
      settings: AttributesFormatString=<initial=%<InitialCondition>>
  alarm : Outport
  timer_value : Outport  Port=2
  wires:
  Logical Operator1/1 -> Logical Operator7/2
  Logical Operator4/1 -> Logical Operator5/2
  target_time/1 -> Switch3/1  "target_time"
  Sum/1 -> Switch2/3
  Unit Delay1/1 -> Logical Operator4/1
  Constant5/1 -> Switch2/1
  Sum1/1 -> Relational Operator/2
  Logical Operator2/1 -> alarm/1  "alarm"
  Constant3/1 -> Sum1/1
  Relational Operator/1 -> Logical Operator2/2
  start_flag/1 -> Logical Operator2/1, Unit Delay1/1, Logical Operator5/1, Logical Operator1/1  "start_flag"
  Switch3/1 -> Relational Operator/1, MinMax/1, Unit Delay2/1  "sampled_target_time"
  Unit Delay2/1 -> Switch3/3
  Switch2/1 -> MinMax/2
  Logical Operator7/1 -> Switch2/2
  Constant1/1 -> Sum/1
  Logical Operator5/1 -> Switch3/2, Logical Operator7/1  "edge"
  Unit Delay/1 -> Sum/2  "timer_value_old"
  MinMax/1 -> timer_value/1, Unit Delay/1, Sum1/2  "timer_value"

== system AEMS_Standard_Library/TIMER/AEMS_TIMER1 ==
  Init : Inport
  Duration : Inport  Port=2
  Timestep : Inport  Port=3
  Constant1 : Constant  Value=0  OutDataTypeStr=single
  Constant2 : Constant  Value=1000  OutDataTypeStr=single
  Constant3 : Constant  Value=1000  OutDataTypeStr=single
  Constant4 : Constant  Value=0  OutDataTypeStr=single
  Constant5 : Constant  Value=1000  OutDataTypeStr=single
  DelayInput1 : UnitDelay  Description=\nStore in Global RAM  InitialCondition=timeoutinit  SampleTime=-1
      settings: AttributesFormatString=IC = %<X0>
  DelayInput2 : UnitDelay  Description=\nStore in Global RAM  SampleTime=-1
      settings: AttributesFormatString=IC = %<X0>
  EdgeRising : Subsystem
  LogicalOperator : Logic  OutDataTypeStr=boolean
  Product1 : Product  OutDataTypeStr=Inherit: Inherit via back propagation  RndMeth=Zero
  Product2 : Product  OutDataTypeStr=Inherit: Inherit via back propagation  RndMeth=Zero
  Product3 : Product  Inputs=*/  OutDataTypeStr=Inherit: Inherit via back propagation  RndMeth=Zero
  RelationalOperator1 : RelationalOperator  OutDataTypeStr=boolean  ZeroCross=off  RndMeth=Nearest  InputSameDT=on
  Sum : Sum  Inputs=+-  OutDataTypeStr=Inherit: Inherit via back propagation  RndMeth=Zero  SaturateOnIntegerOverflow=on  InputSameDT=on
      settings: AttributesFormatString=SAT = %<SaturateOnIntegerOverflow>
  Sum1 : Sum  OutDataTypeStr=Inherit: Inherit via back propagation  RndMeth=Zero  SaturateOnIntegerOverflow=on  InputSameDT=on
      settings: AttributesFormatString=SAT = %<SaturateOnIntegerOverflow>
  Switch1 : Switch  Criteria=u2 ~= 0  RndMeth=Zero  SaturateOnIntegerOverflow=on  InputSameDT=on
      settings: AttributesFormatString=Criteria=%<Criteria>
  Switch2 : Switch  Criteria=u2 ~= 0  RndMeth=Zero  SaturateOnIntegerOverflow=on  InputSameDT=on
      settings: AttributesFormatString=Criteria=%<Criteria>
  Switch3 : Switch  Criteria=u2 ~= 0  RndMeth=Zero  SaturateOnIntegerOverflow=on  InputSameDT=on
      settings: AttributesFormatString=Criteria=%<Criteria>
  Timeout : Outport
  Timer : Outport  Port=2
  wires:
  Switch3/1 -> DelayInput2/1, Product3/1
  Constant1/1 -> Switch3/1
  RelationalOperator1/1 -> Switch3/2, LogicalOperator/2
  Sum1/1 -> Switch2/1
  DelayInput1/1 -> Switch1/3
  Switch1/1 -> LogicalOperator/1, DelayInput1/1  "Flag_of_first_initialisation"
  LogicalOperator/1 -> Timeout/1
  Constant4/1 -> RelationalOperator1/1
  Sum/1 -> RelationalOperator1/2, Switch3/3
  Init/1 -> EdgeRising/1(In)
  Switch2/1 -> Sum/1
  EdgeRising/1(Out) -> Switch1/1, Switch1/2, Switch2/2
  DelayInput2/1 -> Switch2/3
  Product2/1 -> Sum/2, Sum1/2
  Duration/1 -> Product1/1
  Product1/1 -> Sum1/1
  Timestep/1 -> Product2/1
  Constant5/1 -> Product3/2
  Product3/1 -> Timer/1
  Constant3/1 -> Product1/2
  Constant2/1 -> Product2/2

== system AEMS_Standard_Library/TIMER/AEMS_TIMER_H ==
  start_flag : Inport  OutDataTypeStr=boolean
  clear_flag : Inport  Port=2  OutDataTypeStr=boolean
  target_time : Inport  Port=3
  Constant1 : Constant  Value=sample_time  OutDataTypeStr=Inherit: Inherit via back propagation
  Constant3 : Constant  Value=0.0001  OutDataTypeStr=Inherit: Inherit via back propagation
  Constant4 : Constant  Value=0  OutDataTypeStr=Inherit: Inherit via back propagation
  Constant5 : Constant  Value=0  OutDataTypeStr=Inherit: Inherit via back propagation
  Logical Operator2 : Logic  Operator=OR  OutDataTypeStr=boolean
  Logical Operator3 : Logic  OutDataTypeStr=boolean
  Logical Operator4 : Logic  Operator=NOT  OutDataTypeStr=boolean
  Logical Operator5 : Logic  OutDataTypeStr=boolean
  Logical Operator6 : Logic  Operator=NOT  OutDataTypeStr=boolean
  Logical Operator7 : Logic  Operator=OR  OutDataTypeStr=boolean
  Logical Operator8 : Logic  OutDataTypeStr=boolean
  MinMax : MinMax  Inputs=2  SaturateOnIntegerOverflow=on  InputSameDT=on
  Relational Operator : RelationalOperator  Operator=<=  OutDataTypeStr=boolean  RndMeth=Nearest  InputSameDT=on
  Relational Operator1 : RelationalOperator  Operator=<=  OutDataTypeStr=boolean  RndMeth=Nearest  InputSameDT=on
  Sum : Sum  OutDataTypeStr=Inherit: Inherit via back propagation  InputSameDT=on
  Sum1 : Sum  OutDataTypeStr=Inherit: Inherit via back propagation  InputSameDT=on
  Switch{,1..3} (4 alike) : Switch  Criteria=u2 ~= 0  SaturateOnIntegerOverflow=on  InputSameDT=on
      settings: AttributesFormatString=Criteria=%<Criteria>
  Unit Delay{,1..3} (4 alike) : UnitDelay  SampleTime=-1
      settings: AttributesFormatString=<initial=%<InitialCondition>>
  alarm : Outport
  timer_value : Outport  Port=2
  wires:
  Constant5/1 -> Switch2/1
  Sum1/1 -> Relational Operator/2
  Constant4/1 -> Relational Operator1/2
  Switch1/1 -> alarm/1  "alarm"
  Relational Operator1/1 -> Switch1/2  "timer_kill"
  Constant3/1 -> Sum1/1
  Relational Operator/1 -> Switch1/3
  Switch3/1 -> Relational Operator/1, MinMax/1, Unit Delay2/1, Relational Operator1/1  "sampled_target_time"
  Unit Delay2/1 -> Switch3/3
  Switch2/1 -> MinMax/2
  Logical Operator7/1 -> Switch2/2
  Switch/1 -> Switch2/3
  Sum/1 -> Switch/1
  Constant1/1 -> Sum/1
  Logical Operator2/1 -> Logical Operator3/2
  Logical Operator3/1 -> Unit Delay1/1, Logical Operator5/2, Unit Delay3/1, Switch3/2, Switch1/1  "start_to_clear"
  Unit Delay1/1 -> Logical Operator2/2  "start_to_clear_old"
  target_time/1 -> Switch3/1  "target_time"
  Logical Operator6/1 -> Logical Operator3/1, Logical Operator8/1  "not_clear"
  Logical Operator8/1 -> Logical Operator2/1
  clear_flag/1 -> Logical Operator7/2, Logical Operator6/1  "clear_flag"
  Unit Delay/1 -> Sum/2, Switch/3  "timer_value_old"
  MinMax/1 -> timer_value/1, Unit Delay/1, Sum1/2  "timer_value"
  start_flag/1 -> Switch/2, Logical Operator8/2  "start_flag"
  Logical Operator4/1 -> Logical Operator5/1
  Unit Delay3/1 -> Logical Operator4/1
  Logical Operator5/1 -> Logical Operator7/1  "edge"

== system AEMS_Standard_Library/TIMER/AEMS_TURN_OFF_DELAY ==
  Delaytime : Inport  Tag=AM,In,0,1,Name,C;CMP,Port,PortWidth,SampleTime;
  Signal : Inport  Tag=AM,In,0,1,Name,C;CMP,Port,PortWidth,SampleTime;  Port=2
  Timestep : Inport  Tag=AM,In,0,1,Name,C;CMP,Port,PortWidth,SampleTime;  Port=3
  AEMS_TIMER2 : AEMS_Standard_Library/TIMER/AEMS_TIMER1  Tag=[LIB]  timeoutinit=not(timeoutinit)  initinit=not(initinit)
      settings: AttributesFormatString=%<MaskType>\nTimeout output initialisation=%<timeoutinit>\nInit input initialisation=%<initinit>
  Logical_Operator : Logic  Tag=AM,Std,Inputs,1;CMP,Operator,Inputs;  Operator=OR  OutDataTypeStr=boolean
  Logical_Operator1 : Logic  Tag=AM,Std,Inputs,1;CMP,Operator,Inputs;  Operator=NOT  OutDataTypeStr=boolean
  Logical_Operator2 : Logic  Tag=AM,Std,Inputs,1;CMP,Operator,Inputs;  Operator=NOT  OutDataTypeStr=boolean
  Terminator : Terminator
  Out : Outport  Tag=AM,Out,1,0,Name,NC;CMP,Port,OutputWhenDisabled,InitialOutput;
  wires:
  AEMS_TIMER2/2 -> Terminator/1
  AEMS_TIMER2/1 -> Logical_Operator2/1
  Logical_Operator1/1 -> AEMS_TIMER2/1
  Logical_Operator2/1 -> Logical_Operator/2
  Delaytime/1 -> AEMS_TIMER2/2
  Logical_Operator/1 -> Out/1  "Out"
  Signal/1 -> Logical_Operator/1, Logical_Operator1/1
  Timestep/1 -> AEMS_TIMER2/3

== system AEMS_Standard_Library/TIMER/AEMS_TURN_ON_DELAY ==
  Delaytime : Inport  Tag=AM,In,0,1,Name,C;CMP,Port,PortWidth,SampleTime;
  Signal : Inport  Tag=AM,In,0,1,Name,C;CMP,Port,PortWidth,SampleTime;  Port=2
  Timestep : Inport  Tag=AM,In,0,1,Name,C;CMP,Port,PortWidth,SampleTime;  Port=3
  AEMS_TIMER2 : AEMS_Standard_Library/TIMER/AEMS_TIMER1  Tag=[LIB]  timeoutinit=timeoutinit  initinit=initinit
      settings: AttributesFormatString=%<MaskType>\nTimeout output initialisation=%<timeoutinit>\nInit input initialisation=%<initinit>
  LogicalOperator : Logic  Tag=AM,Std,Inputs,1;CMP,Operator,Inputs;  OutDataTypeStr=boolean
  Terminator : Terminator
  Out : Outport  Tag=AM,Out,1,0,Name,NC;CMP,Port,OutputWhenDisabled,InitialOutput;
  wires:
  Timestep/1 -> AEMS_TIMER2/3
  AEMS_TIMER2/1 -> LogicalOperator/2
  LogicalOperator/1 -> Out/1
  Signal/1 -> AEMS_TIMER2/1, LogicalOperator/1  "Signal"
  AEMS_TIMER2/2 -> Terminator/1
  Delaytime/1 -> AEMS_TIMER2/2

== system AEMS_Standard_Library/TRIGGER/AEMS_EVENT ==
  Relational Operator : RelationalOperator  Operator=<  OutDataTypeStr=boolean  RndMeth=Nearest  InputSameDT=on
  Unit Delay : UnitDelay  SampleTime=-1
      settings: AttributesFormatString=<initial=%<X0>>
  imm : Constant  Value=0.0001  OutDataTypeStr=Inherit: Inherit via back propagation
  imm_clear : Constant  Value=0  OutDataTypeStr=Inherit: Inherit via back propagation
  imm_event_time : Constant  Value=event_time  OutDataTypeStr=Inherit: Inherit via back propagation
  imm_sampling_time : Constant  Value=sample_time  OutDataTypeStr=Inherit: Inherit via back propagation
  inclement : Sum  SaturateOnIntegerOverflow=on
  reset : Switch  Threshold=0.5  SaturateOnIntegerOverflow=on  InputSameDT=on
      settings: AttributesFormatString=<threshold=%<threshold>>
  target : Sum  Inputs=++-  SaturateOnIntegerOverflow=on
  event : Outport
  wires:
  imm/1 -> target/2
  Relational Operator/1 -> reset/2, event/1  "event"
  inclement/1 -> reset/3, Relational Operator/2  "timer"
  imm_sampling_time/1 -> target/3, inclement/1  "sample_time"
  target/1 -> Relational Operator/1  "target"
  Unit Delay/1 -> inclement/2
  imm_event_time/1 -> target/1
  imm_clear/1 -> reset/1
  reset/1 -> Unit Delay/1

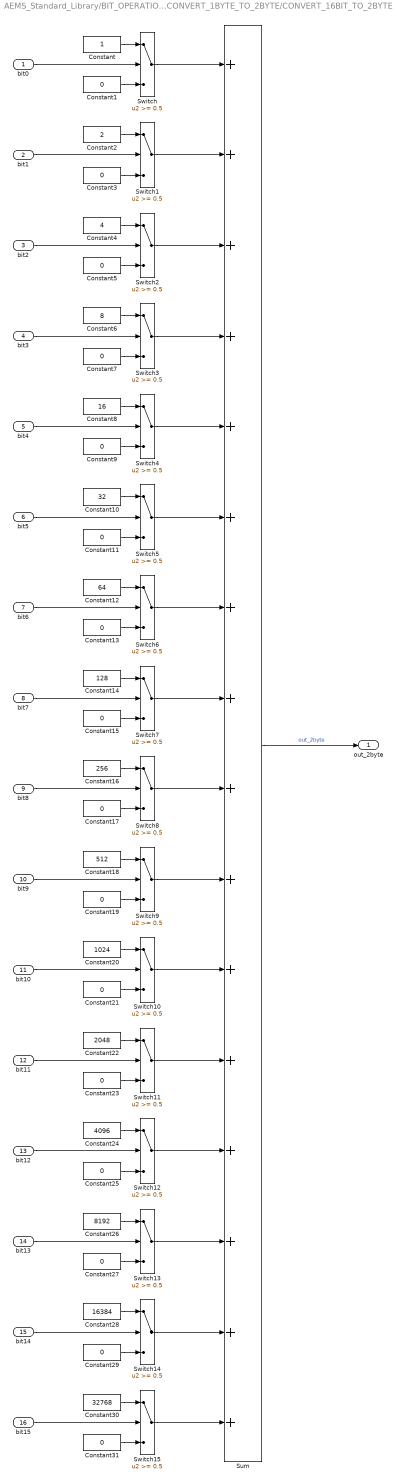
== system AEMS_Standard_Library/BIT_OPERATION/AEMS_CONVERT_1BYTE_TO_2BYTE/CONVERT_16BIT_TO_2BYTE ==
  bit0 : Inport  OutDataTypeStr=boolean  PortDimensions=1
      settings: AttributesFormatString=<tsample=%<SampleTime>>
  bit1 : Inport  Port=2  OutDataTypeStr=boolean  PortDimensions=1
      settings: AttributesFormatString=<tsample=%<SampleTime>>
  bit2 : Inport  Port=3  OutDataTypeStr=boolean  PortDimensions=1
      settings: AttributesFormatString=<tsample=%<SampleTime>>
  bit3 : Inport  Port=4  OutDataTypeStr=boolean  PortDimensions=1
      settings: AttributesFormatString=<tsample=%<SampleTime>>
  bit4 : Inport  Port=5  OutDataTypeStr=boolean  PortDimensions=1
      settings: AttributesFormatString=<tsample=%<SampleTime>>
  bit5 : Inport  Port=6  OutDataTypeStr=boolean  PortDimensions=1
      settings: AttributesFormatString=<tsample=%<SampleTime>>
  bit6 : Inport  Port=7  OutDataTypeStr=boolean  PortDimensions=1
      settings: AttributesFormatString=<tsample=%<SampleTime>>
  bit7 : Inport  Port=8  OutDataTypeStr=boolean  PortDimensions=1
      settings: AttributesFormatString=<tsample=%<SampleTime>>
  bit8 : Inport  Port=9  OutDataTypeStr=boolean  PortDimensions=1
      settings: AttributesFormatString=<tsample=%<SampleTime>>
  bit9 : Inport  Port=10  OutDataTypeStr=boolean  PortDimensions=1
      settings: AttributesFormatString=<tsample=%<SampleTime>>
  bit10 : Inport  Port=11  OutDataTypeStr=boolean  PortDimensions=1
      settings: AttributesFormatString=<tsample=%<SampleTime>>
  bit11 : Inport  Port=12  OutDataTypeStr=boolean  PortDimensions=1
      settings: AttributesFormatString=<tsample=%<SampleTime>>
  bit12 : Inport  Port=13  OutDataTypeStr=boolean  PortDimensions=1
      settings: AttributesFormatString=<tsample=%<SampleTime>>
  bit13 : Inport  Port=14  OutDataTypeStr=boolean  PortDimensions=1
      settings: AttributesFormatString=<tsample=%<SampleTime>>
  bit14 : Inport  Port=15  OutDataTypeStr=boolean  PortDimensions=1
      settings: AttributesFormatString=<tsample=%<SampleTime>>
  bit15 : Inport  Port=16  OutDataTypeStr=boolean  PortDimensions=1
      settings: AttributesFormatString=<tsample=%<SampleTime>>
  Constant : Constant  OutDataTypeStr=uint8
  Constant{1,3,5,7,9,11,13,15} (8 alike) : Constant  Value=0  OutDataTypeStr=uint8
  Constant10 : Constant  Value=32  OutDataTypeStr=uint8
  Constant12 : Constant  Value=64  OutDataTypeStr=uint8
  Constant14 : Constant  Value=128  OutDataTypeStr=uint8
  Constant16 : Constant  Value=256  OutDataTypeStr=uint16
  Constant{17,19,21,23,25,27,29,31} (8 alike) : Constant  Value=0  OutDataTypeStr=uint16
  Constant18 : Constant  Value=512  OutDataTypeStr=uint16
  Constant2 : Constant  Value=2  OutDataTypeStr=uint8
  Constant20 : Constant  Value=1024  OutDataTypeStr=uint16
  Constant22 : Constant  Value=2048  OutDataTypeStr=uint16
  Constant24 : Constant  Value=4096  OutDataTypeStr=uint16
  Constant26 : Constant  Value=8192  OutDataTypeStr=uint16
  Constant28 : Constant  Value=16384  OutDataTypeStr=uint16
  Constant30 : Constant  Value=32768  OutDataTypeStr=uint16
  Constant4 : Constant  Value=4  OutDataTypeStr=uint8
  Constant6 : Constant  Value=8  OutDataTypeStr=uint8
  Constant8 : Constant  Value=16  OutDataTypeStr=uint8
  Sum : Sum  Inputs=16  SaturateOnIntegerOverflow=on
  Switch{,1..15} (16 alike) : Switch  Threshold=0.5  SaturateOnIntegerOverflow=on  InputSameDT=on
      settings: AttributesFormatString=<threshold=%<threshold>>
  out_2byte : Outport
  wires:
  bit8/1 -> Switch8/2
  Constant16/1 -> Switch8/1
  Constant17/1 -> Switch8/3
  bit9/1 -> Switch9/2
  Constant18/1 -> Switch9/1
  Constant19/1 -> Switch9/3
  bit10/1 -> Switch10/2
  Constant20/1 -> Switch10/1
  Constant21/1 -> Switch10/3
  bit11/1 -> Switch11/2
  Constant22/1 -> Switch11/1
  Constant23/1 -> Switch11/3
  bit12/1 -> Switch12/2
  Constant24/1 -> Switch12/1
  Constant25/1 -> Switch12/3
  bit13/1 -> Switch13/2
  Constant26/1 -> Switch13/1
  Constant27/1 -> Switch13/3
  bit14/1 -> Switch14/2
  Constant28/1 -> Switch14/1
  Constant29/1 -> Switch14/3
  bit15/1 -> Switch15/2
  Constant30/1 -> Switch15/1
  Constant31/1 -> Switch15/3
  Switch8/1 -> Sum/9
  Switch9/1 -> Sum/10
  Switch10/1 -> Sum/11
  Switch11/1 -> Sum/12
  Switch12/1 -> Sum/13
  Switch13/1 -> Sum/14
  Switch14/1 -> Sum/15
  Switch15/1 -> Sum/16
  bit0/1 -> Switch/2
  Constant/1 -> Switch/1
  Constant1/1 -> Switch/3
  bit1/1 -> Switch1/2
  Constant2/1 -> Switch1/1
  Constant3/1 -> Switch1/3
  bit2/1 -> Switch2/2
  Constant4/1 -> Switch2/1
  Constant5/1 -> Switch2/3
  bit3/1 -> Switch3/2
  Constant6/1 -> Switch3/1
  Constant7/1 -> Switch3/3
  bit4/1 -> Switch4/2
  Constant8/1 -> Switch4/1
  Constant9/1 -> Switch4/3
  bit5/1 -> Switch5/2
  Constant10/1 -> Switch5/1
  Constant11/1 -> Switch5/3
  bit6/1 -> Switch6/2
  Constant12/1 -> Switch6/1
  Constant13/1 -> Switch6/3
  bit7/1 -> Switch7/2
  Constant14/1 -> Switch7/1
  Constant15/1 -> Switch7/3
  Switch/1 -> Sum/1
  Switch1/1 -> Sum/2
  Switch2/1 -> Sum/3
  Switch3/1 -> Sum/4
  Switch4/1 -> Sum/5
  Switch5/1 -> Sum/6
  Switch6/1 -> Sum/7
  Switch7/1 -> Sum/8
  Sum/1 -> out_2byte/1  "out_2byte"

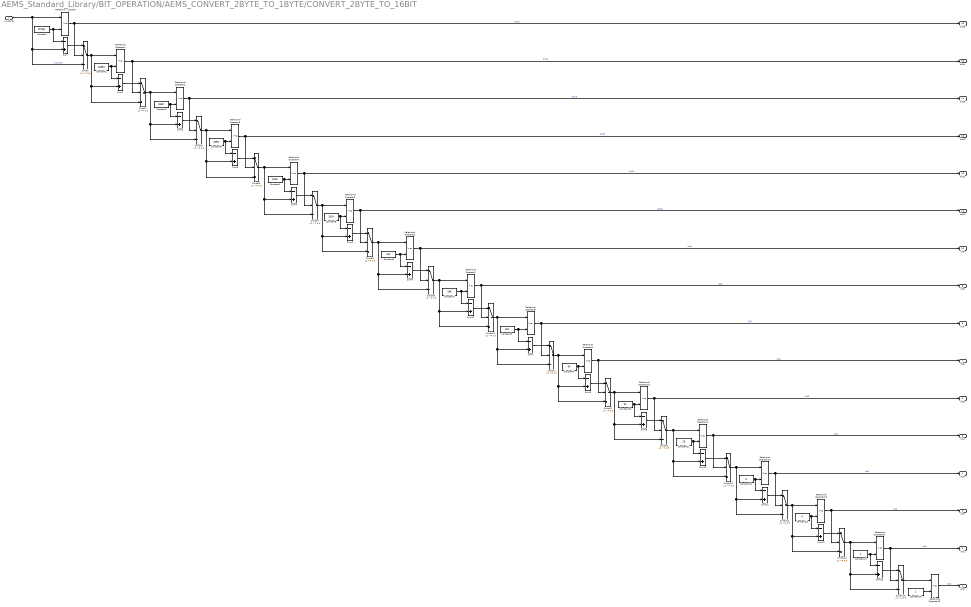
== system AEMS_Standard_Library/BIT_OPERATION/AEMS_CONVERT_2BYTE_TO_1BYTE/CONVERT_2BYTE_TO_16BIT ==
  in_2byte : Inport  OutDataTypeStr=uint16  PortDimensions=1
      settings: AttributesFormatString=<tsample=%<SampleTime>>
  Constant : Constant  Value=32768  OutDataTypeStr=uint16
  Constant1 : Constant  Value=16384  OutDataTypeStr=uint16
  Constant10 : Constant  Value=32  OutDataTypeStr=uint16
  Constant11 : Constant  Value=16  OutDataTypeStr=uint16
  Constant12 : Constant  Value=8  OutDataTypeStr=uint16
  Constant13 : Constant  Value=4  OutDataTypeStr=uint16
  Constant14 : Constant  Value=2  OutDataTypeStr=uint16
  Constant15 : Constant  OutDataTypeStr=uint16
  Constant2 : Constant  Value=8192  OutDataTypeStr=uint16
  Constant3 : Constant  Value=4096  OutDataTypeStr=uint16
  Constant4 : Constant  Value=2048  OutDataTypeStr=uint16
  Constant5 : Constant  Value=1024  OutDataTypeStr=uint16
  Constant6 : Constant  Value=512  OutDataTypeStr=uint16
  Constant7 : Constant  Value=256  OutDataTypeStr=uint16
  Constant8 : Constant  Value=128  OutDataTypeStr=uint16
  Constant9 : Constant  Value=64  OutDataTypeStr=uint16
  Relational Operator{,1..15} (16 alike) : RelationalOperator  OutDataTypeStr=boolean  RndMeth=Nearest  InputSameDT=on
  Sum{,1..14} (15 alike) : Sum  Inputs=-+  SaturateOnIntegerOverflow=on  InputSameDT=on
  Switch{,1..14} (15 alike) : Switch  Threshold=0.5  SaturateOnIntegerOverflow=on  InputSameDT=on
  bit0 : Outport
  bit1 : Outport  Port=2
  bit2 : Outport  Port=3
  bit3 : Outport  Port=4
  bit4 : Outport  Port=5
  bit5 : Outport  Port=6
  bit6 : Outport  Port=7
  bit7 : Outport  Port=8
  bit8 : Outport  Port=9
  bit9 : Outport  Port=10
  bit10 : Outport  Port=11
  bit11 : Outport  Port=12
  bit12 : Outport  Port=13
  bit13 : Outport  Port=14
  bit14 : Outport  Port=15
  bit15 : Outport  Port=16
  wires:
  Switch14/1 -> Switch7/3, Sum7/2, Relational Operator8/1
  Sum14/1 -> Switch14/1
  Constant8/1 -> Sum7/1, Relational Operator8/2
  Relational Operator8/1 -> Switch7/2, bit7/1  "bit7"
  Sum7/1 -> Switch7/1
  Constant9/1 -> Sum8/1, Relational Operator9/2
  Switch7/1 -> Switch8/3, Sum8/2, Relational Operator9/1
  Sum8/1 -> Switch8/1
  Relational Operator9/1 -> Switch8/2, bit6/1  "bit6"
  Constant10/1 -> Relational Operator10/2, Sum9/1
  Sum9/1 -> Switch9/1
  Relational Operator10/1 -> bit5/1, Switch9/2  "bit5"
  Switch8/1 -> Switch9/3, Sum9/2, Relational Operator10/1
  Constant11/1 -> Sum10/1, Relational Operator11/2
  Sum10/1 -> Switch10/1
  Relational Operator11/1 -> Switch10/2, bit4/1  "bit4"
  Switch9/1 -> Switch10/3, Sum10/2, Relational Operator11/1
  Constant12/1 -> Relational Operator12/2, Sum11/1
  Sum11/1 -> Switch11/1
  Relational Operator12/1 -> bit3/1, Switch11/2  "bit3"
  Switch10/1 -> Sum11/2, Switch11/3, Relational Operator12/1
  Constant13/1 -> Sum12/1, Relational Operator13/2
  Sum12/1 -> Switch12/1
  Relational Operator13/1 -> Switch12/2, bit2/1  "bit2"
  Switch11/1 -> Switch12/3, Sum12/2, Relational Operator13/1
  Constant14/1 -> Relational Operator14/2, Sum13/1
  Sum13/1 -> Switch13/1
  Relational Operator14/1 -> bit1/1, Switch13/2  "bit1"
  Switch12/1 -> Switch13/3, Sum13/2, Relational Operator14/1
  Constant15/1 -> Relational Operator15/2
  Switch13/1 -> Relational Operator15/1
  Relational Operator15/1 -> bit0/1  "bit0"
  in_2byte/1 -> Relational Operator/1, Sum/2, Switch/3  "in_2byte"
  Constant/1 -> Relational Operator/2, Sum/1
  Relational Operator/1 -> bit15/1, Switch/2  "bit15"
  Sum/1 -> Switch/1
  Constant1/1 -> Relational Operator1/2, Sum1/1
  Switch/1 -> Relational Operator1/1, Sum1/2, Switch1/3
  Sum1/1 -> Switch1/1
  Relational Operator1/1 -> bit14/1, Switch1/2  "bit14"
  Constant2/1 -> Sum2/1, Relational Operator2/2
  Sum2/1 -> Switch2/1
  Relational Operator2/1 -> Switch2/2, bit13/1  "bit13"
  Switch1/1 -> Relational Operator2/1, Sum2/2, Switch2/3
  Constant3/1 -> Relational Operator3/2, Sum3/1
  Sum3/1 -> Switch3/1
  Relational Operator3/1 -> bit12/1, Switch3/2  "bit12"
  Switch2/1 -> Relational Operator3/1, Sum3/2, Switch3/3
  Constant4/1 -> Sum4/1, Relational Operator4/2
  Sum4/1 -> Switch4/1
  Relational Operator4/1 -> Switch4/2, bit11/1  "bit11"
  Switch3/1 -> Relational Operator4/1, Switch4/3, Sum4/2
  Constant5/1 -> Relational Operator5/2, Sum5/1
  Sum5/1 -> Switch5/1
  Relational Operator5/1 -> bit10/1, Switch5/2  "bit10"
  Switch4/1 -> Relational Operator5/1, Sum5/2, Switch5/3
  Constant6/1 -> Sum6/1, Relational Operator6/2
  Sum6/1 -> Switch6/1
  Relational Operator6/1 -> Switch6/2, bit9/1  "bit9"
  Switch5/1 -> Relational Operator6/1, Sum6/2, Switch6/3
  Constant7/1 -> Sum14/1, Relational Operator7/2
  Switch6/1 -> Sum14/2, Switch14/3, Relational Operator7/1
  Relational Operator7/1 -> Switch14/2, bit8/1  "bit8"
